simulink model "bug_report"  (R2018b)
settings: Solver=FixedStepDiscrete  StartTime=0.0  StopTime=10.0  FixedStep=1  RelTol=1e-3
libraries: slident x2
settings Model: Creator=Trips  LastModifiedBy=Trips
settings ConfigComp: PLC_OutputDir=internal  PLC_TargetIDE=step7  PLC_GenerateReport=off  PLC_LaunchReport=off

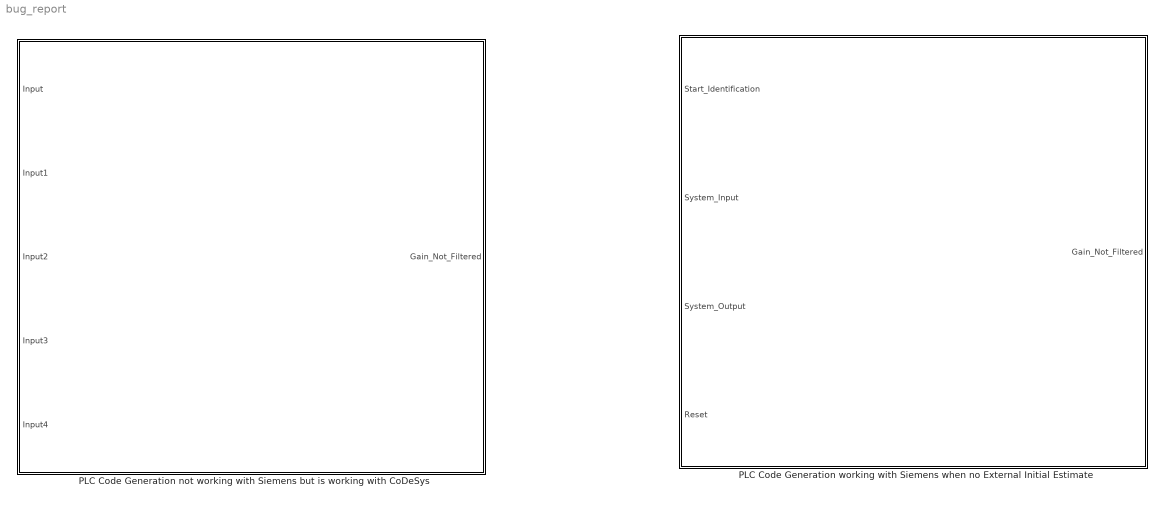
== system bug_report ==
  "PLC Code Generation not working with Siemens but is working with CoDeSys " : Subsystem  TreatAsAtomicUnit=on  SystemSampleTime=1
  "PLC Code Generation working with Siemens when no External Initial Estimate " : Subsystem  TreatAsAtomicUnit=on  SystemSampleTime=1

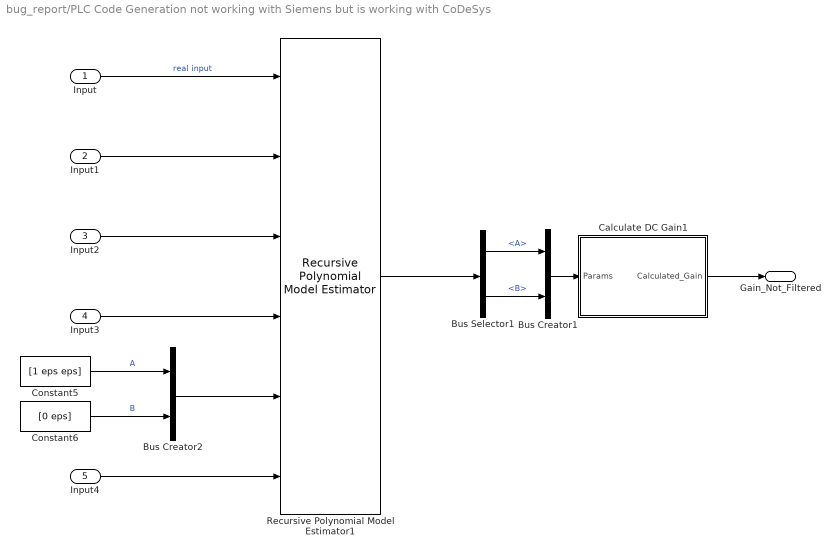
== system bug_report/PLC Code Generation not working with Siemens but is working with CoDeSys  ==
  Input : Inport  SampleTime=1
  Input1 : Inport  Port=2  SampleTime=1
  Input2 : Inport  Port=3  PortDimensions=1  SampleTime=1
  Input3 : Inport  Port=4  PortDimensions=1  SampleTime=1
  Input4 : Inport  Port=5  PortDimensions=1  SampleTime=1
  Bus Creator1 : BusCreator  Inputs=2
  Bus Creator2 : BusCreator  Inputs=2
  Bus Selector1 : BusSelector  OutputSignals=A,B
  Calculate DC Gain1 : Subsystem  TreatAsAtomicUnit=on  SystemSampleTime=1
  Constant5 : Constant  Value=[1 eps eps]  VectorParams1D=off
  Constant6 : Constant  Value=[0 eps]  VectorParams1D=off
  Recursive Polynomial Model Estimator1 : slident/Estimators/Recursive Polynomial Model Estimator  ModelStructure=ARX  InitialEstimateSource=External  A0=2  B0=1  C0=1  D0=1  F0=1  nk=1  P0=100  InitialInputs=0  InitialOutputs=0  History=Infinite  WindowLength=2000  EstimationMethod=Forgetting Factor  AdaptationParameter=1  HasTimeVaryingAdaptationParameter=off  NormalizationBias=eps  OutputError=off  OutputP=off  AddEnablePort=on  ExternalReset=Rising  InputProcessing=Sample-based  Ts=1
      settings: SourceProductName=System Identification Toolbox  SourceProductBaseCode=ID
  Gain_Not_Filtered : Outport
  wires:
  Recursive Polynomial Model Estimator1/1 -> Bus Selector1/1
  Bus Creator1/1 -> Calculate DC Gain1/1(Params)
  Bus Selector1/1 -> Bus Creator1/1  "<A>"
  Bus Selector1/2 -> Bus Creator1/2  "<B>"
  Constant6/1 -> Bus Creator2/2  "B"
  Constant5/1 -> Bus Creator2/1  "A"
  Calculate DC Gain1/1(Calculated_Gain) -> Gain_Not_Filtered/1
  Input/1 -> Recursive Polynomial Model Estimator1/1  "real input"
  Input1/1 -> Recursive Polynomial Model Estimator1/2
  Input2/1 -> Recursive Polynomial Model Estimator1/3
  Bus Creator2/1 -> Recursive Polynomial Model Estimator1/5
  Input4/1 -> Recursive Polynomial Model Estimator1/6
  Input3/1 -> Recursive Polynomial Model Estimator1/4

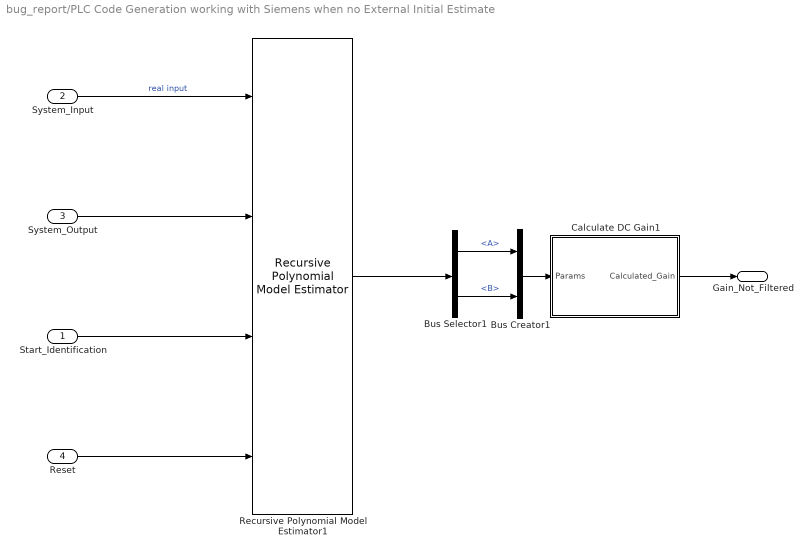
== system bug_report/PLC Code Generation working with Siemens when no External Initial Estimate  ==
  Start_Identification : Inport  SampleTime=1
  System_Input : Inport  Port=2  PortDimensions=1  SampleTime=1
  System_Output : Inport  Port=3  PortDimensions=1  SampleTime=1
  Reset : Inport  Port=4  PortDimensions=1  SampleTime=1
  Bus Creator1 : BusCreator  Inputs=2
  Bus Selector1 : BusSelector  OutputSignals=A,B
  Calculate DC Gain1 : Subsystem  TreatAsAtomicUnit=on  SystemSampleTime=1
  Recursive Polynomial Model Estimator1 : slident/Estimators/Recursive Polynomial Model Estimator  ModelStructure=ARX  InitialEstimateSource=Internal  A0=[1 eps]  B0=[0 eps]  C0=1  D0=1  F0=1  nk=1  P0=100  InitialInputs=0  InitialOutputs=0  History=Infinite  WindowLength=2000  EstimationMethod=Forgetting Factor  AdaptationParameter=1  HasTimeVaryingAdaptationParameter=off  NormalizationBias=eps  OutputError=off  OutputP=off  AddEnablePort=on  ExternalReset=Rising  InputProcessing=Sample-based  Ts=1
      settings: SourceProductName=System Identification Toolbox  SourceProductBaseCode=ID
  Gain_Not_Filtered : Outport
  wires:
  Recursive Polynomial Model Estimator1/1 -> Bus Selector1/1
  Bus Creator1/1 -> Calculate DC Gain1/1(Params)
  Bus Selector1/1 -> Bus Creator1/1  "<A>"
  Bus Selector1/2 -> Bus Creator1/2  "<B>"
  Calculate DC Gain1/1(Calculated_Gain) -> Gain_Not_Filtered/1
  System_Input/1 -> Recursive Polynomial Model Estimator1/1  "real input"
  System_Output/1 -> Recursive Polynomial Model Estimator1/2
  Start_Identification/1 -> Recursive Polynomial Model Estimator1/3
  Reset/1 -> Recursive Polynomial Model Estimator1/4

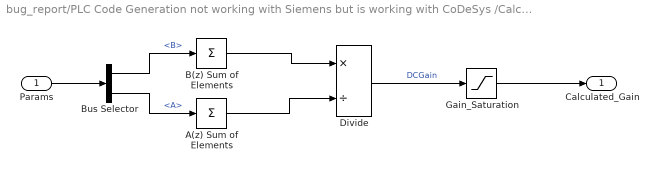
== system bug_report/PLC Code Generation not working with Siemens but is working with CoDeSys /Calculate DC Gain1 ==
  Params : Inport
  A(z) Sum of Elements : Sum  Inputs=+
  B(z) Sum of Elements : Sum  Inputs=+
  Bus Selector : BusSelector  OutputSignals=B,A
  Divide : Product  Inputs=*/
  Gain_Saturation : Saturate  UpperLimit=1.5  LowerLimit=0.01
  Calculated_Gain : Outport
  wires:
  Params/1 -> Bus Selector/1
  Bus Selector/1 -> B(z) Sum of Elements/1  "<B>"
  Bus Selector/2 -> A(z) Sum of Elements/1  "<A>"
  B(z) Sum of Elements/1 -> Divide/1
  Divide/1 -> Gain_Saturation/1  "DCGain"
  A(z) Sum of Elements/1 -> Divide/2
  Gain_Saturation/1 -> Calculated_Gain/1

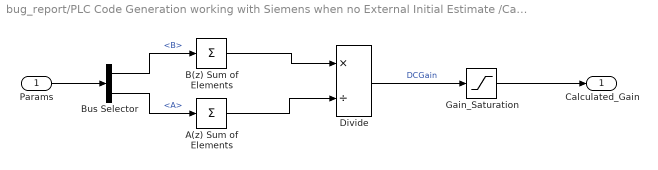
== system bug_report/PLC Code Generation working with Siemens when no External Initial Estimate /Calculate DC Gain1 ==
  Params : Inport
  A(z) Sum of Elements : Sum  Inputs=+
  B(z) Sum of Elements : Sum  Inputs=+
  Bus Selector : BusSelector  OutputSignals=B,A
  Divide : Product  Inputs=*/
  Gain_Saturation : Saturate  UpperLimit=1.5  LowerLimit=0.01
  Calculated_Gain : Outport
  wires:
  Params/1 -> Bus Selector/1
  Bus Selector/1 -> B(z) Sum of Elements/1  "<B>"
  Bus Selector/2 -> A(z) Sum of Elements/1  "<A>"
  B(z) Sum of Elements/1 -> Divide/1
  Divide/1 -> Gain_Saturation/1  "DCGain"
  A(z) Sum of Elements/1 -> Divide/2
  Gain_Saturation/1 -> Calculated_Gain/1
